simulink model "sensorExpoler"  (R2026a)
settings: Solver=FixedStepDiscrete  StopTime=inf  FixedStep=0.001
undefined symbols (not defined in the file): Blocking, Non
libraries: amg_usbconverter_n_connect_lib x2
settings Model: Creator=pboon  LastModifiedBy=mijuuu

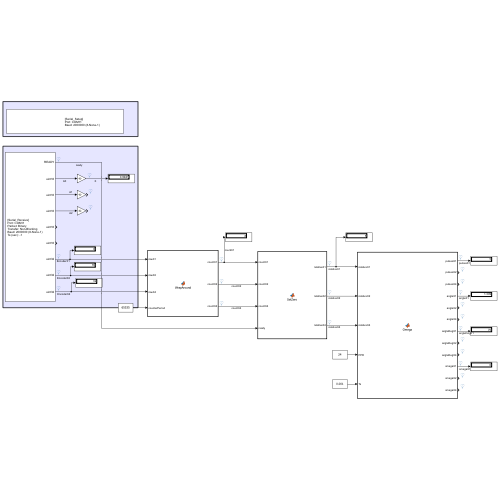
[thumbnail: Simulink's stored preview of the top-level diagram]
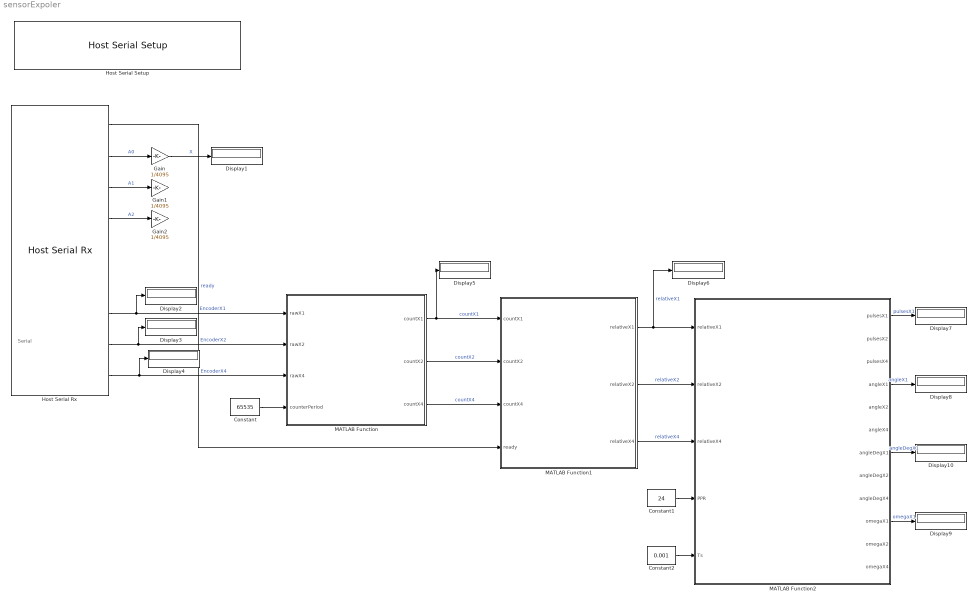
== system sensorExpoler ==
  note: Serial
  Constant : Constant  Value=65535
  Constant1 : Constant  Value=24
  Constant2 : Constant  Value=0.001
  Display{1..10} (10 alike) : Display
  Gain : Gain  Gain=1/4095
  Gain1 : Gain  Gain=1/4095
  Gain2 : Gain  Gain=1/4095
  Host Serial Rx : amg_usbconverter_n_connect_lib/Host Serial Rx  conf=rx  port=<auto>  baudrate=2000000  databits=8  parity=None  stopbit=1  flowcontrol=None  transfer=Non-Blocking  timeout=5  packetmode=Binary  enableinitialvalues=off  initialvalues=[]  binheader='25'  binterminator='4E 4E'  porttype_double=0  porttype_single=0  porttype_int8=0  porttype_uint8=0  porttype_int16=0  porttype_uint16=5  porttype_int32=0  porttype_uint32=3  asciiformat='%d,%f'  rx_asciiterminator="CRLF (0x0D 0x0A - \"\\r\\n\")"  tx_asciiterminator="CRLF (0x0D 0x0A - \"\\r\\n\")"  sampletime=0.001  enablecustomportlabel=off  cinputportlabel=0  coutputportlabel=A  portpinstr=0  blockid=HostSerialRx  inputporttype=[]  inputportwidth=[]  inputportlabel={}  outputporttype=[3 5 5 5 5 5 7 7 7]  outputportwidth=[1 1 1 1 1 1 1 1 1]  outputportlabel={'READY','uint16','uint16','uint16','uint16','uint16','uint32','uint32','uint32'}  compat=0  optionstring=[]  autoport='COM11'
  Host Serial Setup : amg_usbconverter_n_connect_lib/Host Serial Setup  conf=setup  port=<auto>  baudrate=2000000  databits=8  parity=None  stopbit=1  flowcontrol=None  transfer=Blocking  timeout=2  packetmode=Binary  initialvalues=[]  binheader='7E 7E'  binterminator='03 03'  porttype_double=0  porttype_single=1  porttype_int8=0  porttype_uint8=0  porttype_int16=0  porttype_uint16=0  porttype_int32=0  porttype_uint32=2  asciiformat='%d %u %x'  rx_asciiterminator="CRLF (0x0D 0x0A - \"\\r\\n\")"  tx_asciiterminator="CRLF (0x0D 0x0A - \"\\r\\n\")"  sampletime=-1  enablecustomportlabel=off  cinputportlabel=0  coutputportlabel=A  portpinstr=0  blockid=HostSerialSetup  inputporttype=[]  inputportwidth=[]  inputportlabel={}  outputporttype=[]  outputportwidth=[]  outputportlabel={}  compat=0  optionstring=[]  autoport='COM11'
  MATLAB Function : MATLAB Function  TreatAsAtomicUnit=on
  MATLAB Function1 : MATLAB Function  TreatAsAtomicUnit=on
  MATLAB Function2 : MATLAB Function  TreatAsAtomicUnit=on
  wires:
  Host Serial Rx/2 -> Gain/1  "A0"
  Host Serial Rx/3 -> Gain1/1  "A1"
  Host Serial Rx/4 -> Gain2/1  "A2"
  Host Serial Rx/7 -> Display2/1, MATLAB Function/1(rawX1)  "EncoderX1"
  Host Serial Rx/8 -> Display3/1, MATLAB Function/2(rawX2)  "EncoderX2"
  Host Serial Rx/9 -> MATLAB Function/3(rawX4), Display4/1  "EncoderX4"
  Gain/1 -> Display1/1  "X"
  Constant/1 -> MATLAB Function/4(counterPeriod)
  MATLAB Function/1(countX1) -> Display5/1, MATLAB Function1/1(countX1)  "countX1"
  MATLAB Function/3(countX4) -> MATLAB Function1/3(countX4)  "countX4"
  MATLAB Function/2(countX2) -> MATLAB Function1/2(countX2)  "countX2"
  MATLAB Function1/1(relativeX1) -> Display6/1, MATLAB Function2/1(relativeX1)  "relativeX1"
  MATLAB Function1/2(relativeX2) -> MATLAB Function2/2(relativeX2)  "relativeX2"
  MATLAB Function1/3(relativeX4) -> MATLAB Function2/3(relativeX4)  "relativeX4"
  Constant1/1 -> MATLAB Function2/4(PPR)
  Constant2/1 -> MATLAB Function2/5(Ts)
  MATLAB Function2/1(pulsesX1) -> Display7/1  "pulsesX1"
  MATLAB Function2/10(omegaX1) -> Display9/1  "omegaX1"
  MATLAB Function2/4(angleX1) -> Display8/1  "angleX1"
  Host Serial Rx/1 -> MATLAB Function1/4(ready)  "ready"
  MATLAB Function2/7(angleDegX1) -> Display10/1  "angleDegX1"

== matlab function sensorExpoler/MATLAB Function1 ==
  data: countX1 input; countX2 input; countX4 input; relativeX1 output; relativeX2 output; relativeX4 output; ready input
function [relativeX1, relativeX2, relativeX4] = ...
    SetZero(countX1, countX2, countX4, ready)

persistent initialCount savedRelative initialized

if isempty(initialCount)
    initialCount  = zeros(3,1);
    savedRelative = zeros(3,1);
    initialized   = false;
end

% ใช้ข้อมูลเมื่อรับสำเร็จเท่านั้น
if ready ~= 0
    count = [double(countX1);
             double(countX2);
             double(countX4)];

    % ตั้งศูนย์จากข้อมูลจริงครั้งแรก
    if ~initialized
        initialCount = count;
        initialized = true;
    end

    savedRelative = count - initialCount;
end

relativeX1 = savedRelative(1);
relativeX2 = savedRelative(2);
relativeX4 = savedRelative(3);
end

== matlab function sensorExpoler/MATLAB Function ==
  data: rawX1 input; rawX2 input; rawX4 input; countX1 output; counterPeriod input; countX2 output; countX4 output
function [countX1, countX2, countX4] = ...
    WrapAround(rawX1, rawX2, rawX4, counterPeriod)

persistent previousRaw accumulatedCount firstSample

if isempty(previousRaw)
    previousRaw      = zeros(3,1);
    accumulatedCount = zeros(3,1);
    firstSample      = true;
end

raw = [double(rawX1);
       double(rawX2);
       double(rawX4)];

modulus = double(counterPeriod) + 1;

if firstSample
    accumulatedCount = raw;
    firstSample = false;
else
    delta = raw - previousRaw;

    % แก้การข้ามขอบ Counter ทั้งสองทิศทาง
    delta = mod(delta + modulus/2, modulus) - modulus/2;

    accumulatedCount = accumulatedCount + delta;
end

previousRaw = raw;

countX1 = accumulatedCount(1);
countX2 = accumulatedCount(2);
countX4 = accumulatedCount(3);
end

== matlab function sensorExpoler/MATLAB Function2 ==
  data: relativeX1 input; relativeX2 input; relativeX4 input; pulsesX1 output; pulsesX2 output; pulsesX4 output; PPR input; Ts input; angleX1 output; angleX2 output; angleX4 output; angleDegX1 output; angleDegX2 output; angleDegX4 output; omegaX1 output; omegaX2 output; omegaX4 output
function [pulsesX1, pulsesX2, pulsesX4, ...
          angleX1, angleX2, angleX4, ...
          angleDegX1, angleDegX2, angleDegX4, ...
          omegaX1, omegaX2, omegaX4] = ...
    Omega(relativeX1, relativeX2, relativeX4, PPR, Ts)

persistent previousAngle firstSample

if isempty(previousAngle)
    previousAngle = zeros(3,1);
    firstSample   = true;
end

relativeCount = [double(relativeX1);
                 double(relativeX2);
                 double(relativeX4)];

modeFactor = [1; 2; 4];

% Relative Position หน่วย Pulses
pulses = relativeCount ./ modeFactor;

% Angular Position หน่วย rad
angle = pulses .* (2*pi / double(PPR));

% Angular Velocity หน่วย rad/s
if firstSample
    omega = zeros(3,1);
    firstSample = false;
else
    omega = (angle - previousAngle) ./ double(Ts);
end

previousAngle = angle;

pulsesX1 = pulses(1);
pulsesX2 = pulses(2);
pulsesX4 = pulses(3);

angleX1 = angle(1);
angleX2 = angle(2);
angleX4 = angle(3);

angleDegX1 = angleX1 * 180/pi;
angleDegX2 = angleX2 * 180/pi;
angleDegX4 = angleX4 * 180/pi;

omegaX1 = omega(1);
omegaX2 = omega(2);
omegaX4 = omega(3);
end
